simulink library "LSSFunctionLibrary"  (R2019b)
settings: Solver=ode1  StartTime=0.0  StopTime=Inf  FixedStep=0.001  RelTol=1e-3  EnableMultiTasking=on
PostLoadFcn:
  | , if any(exist('dsrtsu_mdlpostloadfcn', 'file') == [2, 3, 6]), try dsrtsu_mdlpostloadfcn('Execute', bdroot); catch fprintf('Error in PostLoadFcn (dsrtsu_mdlpostloadfcn) for model "%s":\n %s\n', bdroot, lasterr); end, end,
undefined symbols (not defined in the file): P_A1_comp_max, P_allow_lane_center_fade, P_assumed_lane_width, P_enable_A1_comp, P_invalid_lane_width_jump_limit, P_Lane_A0_Conf_Limit, P_LCC_STC_AntiWindup_Limit, P_long_dist_camera_to_tire, P_Max_Lane_Width
libraries: $bdroot x1, simulink x1
settings Model: DSRTSU_INTERNAL_RTI_VER=500  DSRTSU_INTERNAL_RTI_TYPE=rti1401  TLRevision=101  RTICANMMDATA=struct('GeneralSetupData',struct('modelroot','C:\WORK\34_GAC\3_A12\A12_H_P\CS322\99999088_GAC_A12P_L2P_Feature_Release\GAC_A12P\DelphiCoreLib\Lateral_Control\ELK','generalsettings',struct('filesettings',struct('destfolder',struct('Name','RTICANMM_FILES','Check',1),'buildfolder',struct('Name','.','Check',1),'AbsDestfolder',struct('Name','C:\WORK\34_GAC\3_A12\A12_H_P\CS322\99999088_GAC_A12P_L2P_Feature_Release\GAC_A12P\DelphiCoreLib\Lateral_Control\ELK\RTICANMM_FILES'),'AbsBuildfolder',struct('Name','C:\WORK\34_GAC\3_A12\A12_H_P\CS322\99999088_GAC_A12P_L2P_Feature_Release\GAC_A12P\DelphiCoreLib\Lateral_Control\ELK'))),'options',struct('addpaths',1,'rmpaths',1,'addtrcexclusion',logical(1),'cannavigator',struct('checkmonitoring',0),'show_usrtrc',0,'use_usrtrc',0),'advanced',struct('options',ones(1,100)),'MPSetup',{{}},'modelname','ELK_fcns_lib','block','ELK_fcns_lib'))  DSRTSU_INTERNAL_RTIFLEXRAYCONFIG=110  DSRTSU_INTERNAL_RTIFPGA=90  Creator=bzxk5y  LastModifiedBy=86156
settings DataIOCC: LimitDataPoints=on  SaveFormat=Array  SignalLoggingSaveFormat=ModelDataLogs  ReturnWorkspaceOutputs=off
settings OptimizationCC: BlockReduction=off  OptimizeBlockIOStorage=off  BufferReuse=off  GlobalBufferReuse=off  ExpressionFolding=off  ExpressionDepthLimit=2147483647  LocalBlockOutputs=off  LifeSpan=inf
settings DebuggingCC: UnderspecifiedInitializationDetection=Classic  MergeDetectMultiDrivingBlocksExec=none  SolverPrmCheckMsg=warning  FcnCallInpInsideContextMsg=warning  AllowSymbolicDim=off  StateNameClashWarn=warning  SFUnexpectedBacktrackingDiag=warning  SFNoUnconditionalDefaultTransitionDiag=warning  SFExecutionAtInitializationDiag=none  ArithmeticOperatorsInVariantConditions=warning
settings HardwareCC: ProdBitPerPointer=32  ProdBitPerSizeT=32  ProdBitPerPtrDiffT=32  ProdLargestAtomicFloat=None  ProdEndianess=BigEndian  ProdWordSize=32  ProdHWDeviceType=Generic->Custom  TargetIntDivRoundTo=Zero  TargetEndianess=BigEndian  TargetHWDeviceType=Generic->Custom
settings ModelReferenceCC: PropagateSignalLabelsOutOfModel=off
settings SFSimCC: SimUseLocalCustomCode=off  CustomCodeUndefinedFunction=UseInterfaceOnly
settings RTWCC: Description=dSPACE DS1401 Hardware Platform  SystemTargetFile=rti1401.tlc  MakeCommand=make_rti  TemplateMakefile=rti1401.tmf  RTWUseLocalCustomCode=off
settings CodeAppCC: StateflowObjectComments=on
settings STFCustomTargetCC: ParMdlRefBuildCompliant=on  MatFileLogging=on  CPPClassGenCompliant=on  SystemTargetFile=rti1401.tlc
settings GRTTargetCC: TargetLangStandard=C89/C90 (ANSI)  CompOptLevelCompliant=off  ConcurrentExecutionCompliant=off  CombineOutputUpdateFcns=off  UseToolchainInfoCompliant=off  ExtModeMexFile=noextcomm
settings ConfigComp: CovMetricSettings=dw  CovSaveCumulativeToWorkspaceVar=on  CovSaveSingleToWorkspaceVar=on  CovExternalEMLEnable=off

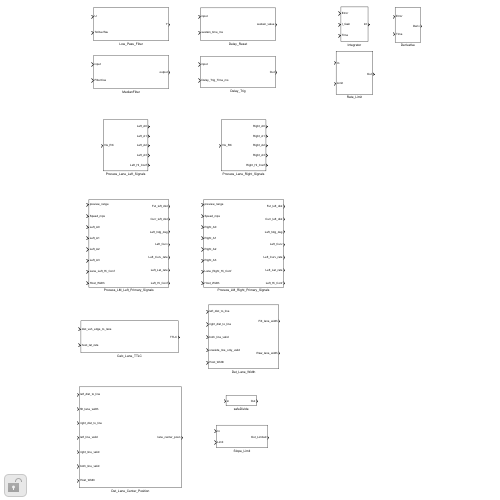
[thumbnail: Simulink's stored preview of the top-level diagram]
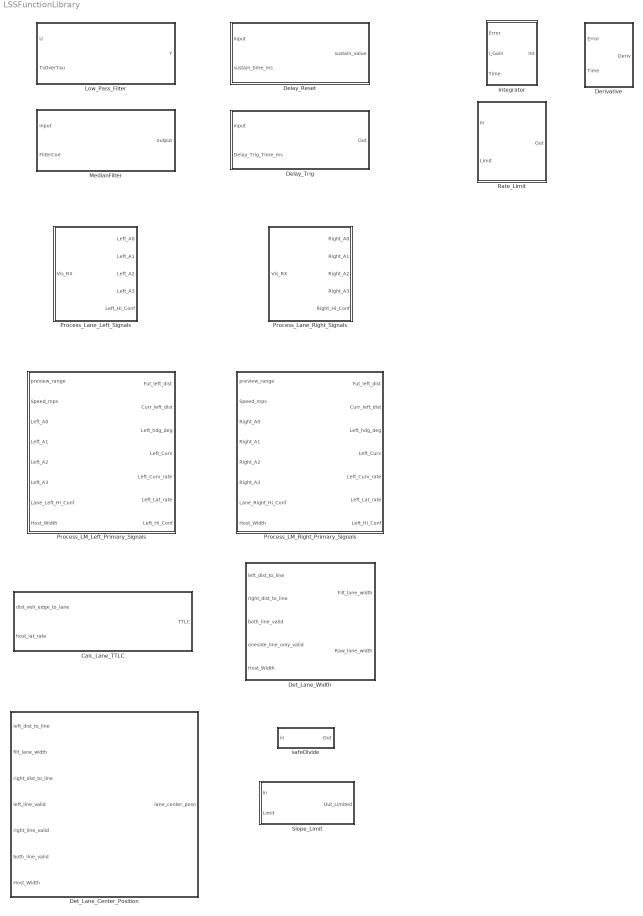
== system LSSFunctionLibrary ==
  Calc_Lane_TTLC : Subsystem
  Delay_Reset : Subsystem
  Delay_Trig : Subsystem
  Derivative : Subsystem
  Det_Lane_Center_Position : Subsystem
  Det_Lane_Width : Subsystem
  Integrator : Subsystem
  Low_Pass_Filter : Subsystem
  MedianFilter : Subsystem
  Process_LM_Left_Primary_Signals : Subsystem
  Process_LM_Right_Primary_Signals : Subsystem
  Process_Lane_Left_Signals : Subsystem
  Process_Lane_Right_Signals : Subsystem
  Rate_Limit : Subsystem
  Slope_Limit : Subsystem
  safeDivide : Subsystem

== system LSSFunctionLibrary/Calc_Lane_TTLC ==
  dist_veh_edge_to_lane : Inport  OutDataTypeStr=single
  host_lat_rate : Inport  Port=2  OutDataTypeStr=single
  Constant : Constant  Value=0.001  OutDataTypeStr=single
  Divide : Product  Inputs=*/  OutDataTypeStr=single
  Max : MinMax  Function=max  Inputs=2  OutDataTypeStr=single
  Saturation : Saturate  UpperLimit=10  LowerLimit=0  OutDataTypeStr=single
  TTLC : Outport  OutDataTypeStr=single
  wires:
  dist_veh_edge_to_lane/1 -> Divide/1
  Max/1 -> Divide/2
  host_lat_rate/1 -> Max/1
  Constant/1 -> Max/2
  Divide/1 -> Saturation/1
  Saturation/1 -> TTLC/1

== system LSSFunctionLibrary/Delay_Reset ==
  input : Inport  Description=_GWMAB30P4.LKAFN.000_316_
  sustain_time_ms : Inport  Description=_GWMAB30P4.LKAFN.000_317_  Port=2
  Sustain_wo_reset : Stateflow chart  Description=_GWMAB30P4.LKAFN.000_319_  TreatAsAtomicUnit=on
  sustain_value : Outport  Description=_GWMAB30P4.LKAFN.000_323_
  wires:
  Sustain_wo_reset/1(sustain_value) -> sustain_value/1
  input/1 -> Sustain_wo_reset/1(input)
  sustain_time_ms/1 -> Sustain_wo_reset/2(sustain_time)

== system LSSFunctionLibrary/Delay_Trig ==
  input : Inport  Description=_GWMAB30P4.LKAFN.000_316_
  Delay_Trig_Time_ms : Inport  Description=_GWMH9P3.LCKFN.000_19_  Port=2
  Delay_Trig : Stateflow chart  TreatAsAtomicUnit=on
  Out : Outport  Description=_GWMH9P3.LCKFN.000_23_
  wires:
  input/1 -> Delay_Trig/1(Input)
  Delay_Trig_Time_ms/1 -> Delay_Trig/2(Delay_Trig_Time)
  Delay_Trig/1(Delay_Trig) -> Out/1

== system LSSFunctionLibrary/Derivative ==
  Error : Inport
  Time : Inport  Port=2
  Delay : Delay  DelayLength=1  InitialCondition=0
  Divide : Product  Inputs=*/
  Sum3 : Sum  Inputs=+-
  Deriv : Outport
  wires:
  Sum3/1 -> Divide/1
  Error/1 -> Delay/1, Sum3/1
  Divide/1 -> Deriv/1  "STC_Error_Derivative"
  Delay/1 -> Sum3/2
  Time/1 -> Divide/2

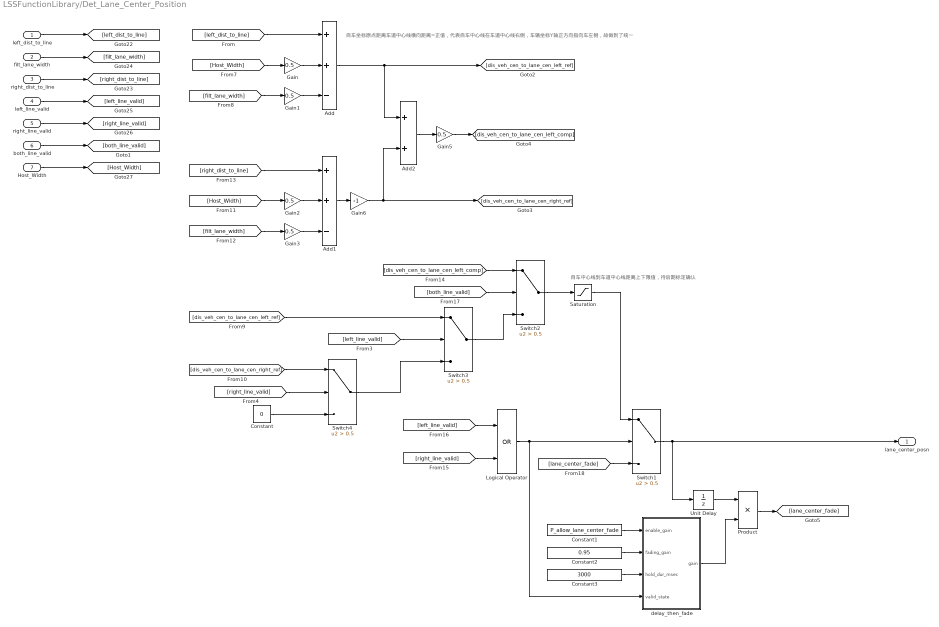
== system LSSFunctionLibrary/Det_Lane_Center_Position ==
  note: 自车中心线到车道中心线距离上下限值，待后期标定确认
  note: 自车坐标原点距离车道中心线横向距离=正值，代表自车中心线在车道中心线右侧，车辆坐标Y轴正方向指向车左侧，故做到了统一
  left_dist_to_line : Inport  OutDataTypeStr=single
  filt_lane_width : Inport  Port=2  OutDataTypeStr=single
  right_dist_to_line : Inport  Port=3  OutDataTypeStr=single
  left_line_valid : Inport  Port=4
  right_line_valid : Inport  Port=5
  both_line_valid : Inport  Port=6
  Host_Width : Inport  Port=7  OutDataTypeStr=single
  Add : Sum  Inputs=++-  OutDataTypeStr=single  AccumDataTypeStr=single
  Add1 : Sum  Inputs=++-  OutDataTypeStr=single  AccumDataTypeStr=single
  Add2 : Sum  OutDataTypeStr=single  AccumDataTypeStr=single
  Constant : Constant  Value=0  OutDataTypeStr=single
  Constant1 : Constant  Value=P_allow_lane_center_fade  OutDataTypeStr=single
  Constant2 : Constant  Value=0.95  OutDataTypeStr=double
  Constant3 : Constant  Value=3000  OutDataTypeStr=single
  Gain{,1..3,5} (5 alike) : Gain  Gain=0.5  OutDataTypeStr=single
  Gain6 : Gain  Gain=-1  OutDataTypeStr=single
  Logical Operator : Logic  Operator=OR  AllPortsSameDT=off  OutDataTypeStr=boolean
  Product : Product  OutDataTypeStr=single
  Saturation : Saturate  UpperLimit=3.5  LowerLimit=-3.5  OutDataTypeStr=single
  Switch{1..4} (4 alike) : Switch  Criteria=u2 > Threshold  Threshold=0.5  OutDataTypeStr=single
  Unit Delay : UnitDelay  SampleTime=-1  HasFrameUpgradeWarning=on
  delay_then_fade : Stateflow chart  TreatAsAtomicUnit=on
  lane_center_posn : Outport  OutDataTypeStr=single
  wires:
  left_dist_to_line/1 -> [left_dist_to_line]
  filt_lane_width/1 -> [filt_lane_width]
  right_dist_to_line/1 -> [right_dist_to_line]
  left_line_valid/1 -> [left_line_valid]
  right_line_valid/1 -> [right_line_valid]
  Host_Width/1 -> [Host_Width]
  [left_dist_to_line] -> Add/1
  both_line_valid/1 -> [both_line_valid]
  [Host_Width] -> Gain/1
  Gain/1 -> Add/2
  Gain1/1 -> Add/3
  [filt_lane_width] -> Gain1/1
  Gain3/1 -> Add1/3
  Gain2/1 -> Add1/2
  [Host_Width] -> Gain2/1
  [right_dist_to_line] -> Add1/1
  [filt_lane_width] -> Gain3/1
  Add/1 -> Add2/1, [dis_veh_cen_to_lane_cen_left_ref]
  Add1/1 -> Gain6/1
  Add2/1 -> Gain5/1
  Gain5/1 -> [dis_veh_cen_to_lane_cen_left_comp]
  [left_line_valid] -> Logical Operator/1
  [right_line_valid] -> Logical Operator/2
  [both_line_valid] -> Switch2/2
  Switch2/1 -> Saturation/1
  [dis_veh_cen_to_lane_cen_left_comp] -> Switch2/1
  Switch3/1 -> Switch2/3
  [left_line_valid] -> Switch3/2
  [dis_veh_cen_to_lane_cen_left_ref] -> Switch3/1
  Switch4/1 -> Switch3/3
  [right_line_valid] -> Switch4/2
  [dis_veh_cen_to_lane_cen_right_ref] -> Switch4/1
  Constant/1 -> Switch4/3
  Switch1/1 -> Unit Delay/1, lane_center_posn/1
  Constant1/1 -> delay_then_fade/1(enable_gain)
  Constant2/1 -> delay_then_fade/2(fading_gain)
  Constant3/1 -> delay_then_fade/3(hold_dur_msec)
  Logical Operator/1 -> delay_then_fade/4(valid_state), Switch1/2
  Unit Delay/1 -> Product/1
  delay_then_fade/1(gain) -> Product/2
  Product/1 -> [lane_center_fade]
  [lane_center_fade] -> Switch1/3
  Saturation/1 -> Switch1/1
  Gain6/1 -> Add2/2, [dis_veh_cen_to_lane_cen_right_ref]

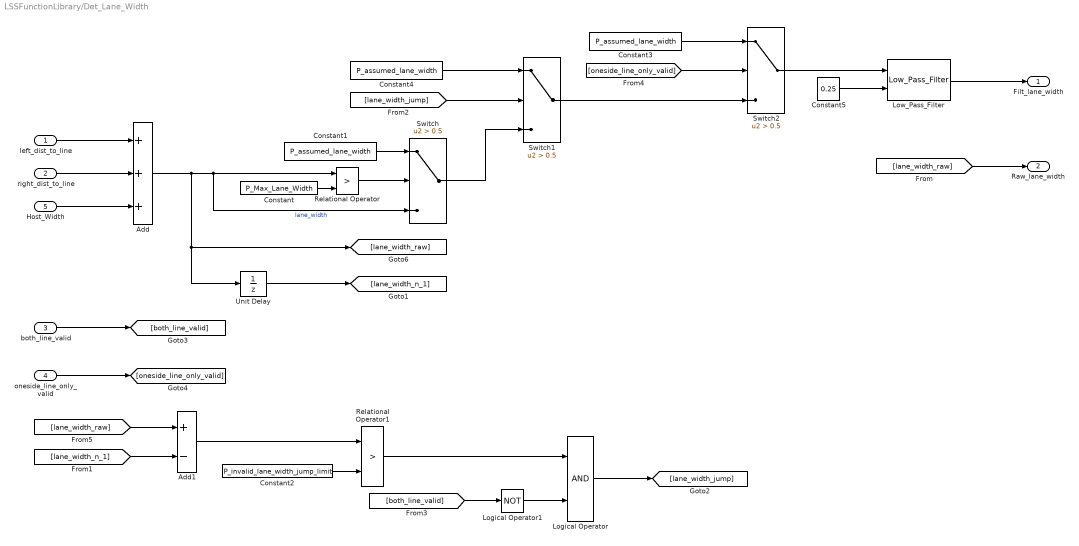
== system LSSFunctionLibrary/Det_Lane_Width ==
  left_dist_to_line : Inport  OutDataTypeStr=single
  right_dist_to_line : Inport  Port=2  OutDataTypeStr=single
  both_line_valid : Inport  Port=3
  oneside_line_only_valid : Inport  Port=4
  Host_Width : Inport  Port=5  OutDataTypeStr=single
  Add : Sum  Inputs=+++  OutDataTypeStr=single  AccumDataTypeStr=single
  Add1 : Sum  Inputs=+-  OutDataTypeStr=single  AccumDataTypeStr=single
  Constant : Constant  Value=P_Max_Lane_Width  OutDataTypeStr=single
  Constant1 : Constant  Value=P_assumed_lane_width  OutDataTypeStr=single
  Constant2 : Constant  Value=P_invalid_lane_width_jump_limit  OutDataTypeStr=single
  Constant3 : Constant  Value=P_assumed_lane_width  OutDataTypeStr=single
  Constant4 : Constant  Value=P_assumed_lane_width  OutDataTypeStr=single
  Constant5 : Constant  Value=0.25  OutDataTypeStr=single
  Logical Operator : Logic  AllPortsSameDT=off  OutDataTypeStr=boolean
  Logical Operator1 : Logic  Operator=NOT  AllPortsSameDT=off  OutDataTypeStr=boolean
  Low_Pass_Filter : $bdroot/Low_Pass_Filter  SystemSampleTime=-1  Latency=0  AutoFrameSizeCalculation=off
  Relational Operator : RelationalOperator  Operator=>  OutDataTypeStr=boolean  RndMeth=Simplest
  Relational Operator1 : RelationalOperator  Operator=>  OutDataTypeStr=boolean  RndMeth=Simplest
  Switch : Switch  Criteria=u2 > Threshold  Threshold=0.5  OutDataTypeStr=single
  Switch1 : Switch  Criteria=u2 > Threshold  Threshold=0.5  OutDataTypeStr=single
  Switch2 : Switch  Criteria=u2 > Threshold  Threshold=0.5  OutDataTypeStr=single
  Unit Delay : UnitDelay  SampleTime=-1  HasFrameUpgradeWarning=on
  Filt_lane_width : Outport  OutDataTypeStr=single
  Raw_lane_width : Outport  Port=2  OutDataTypeStr=single
  wires:
  right_dist_to_line/1 -> Add/2
  left_dist_to_line/1 -> Add/1
  Host_Width/1 -> Add/3
  Add/1 -> Unit Delay/1, [lane_width_raw], Switch/3, Relational Operator/1  "lane_width"
  Constant/1 -> Relational Operator/2
  Relational Operator/1 -> Switch/2
  Constant1/1 -> Switch/1
  Unit Delay/1 -> [lane_width_n_1]
  [lane_width_raw] -> Add1/1
  [lane_width_n_1] -> Add1/2
  Add1/1 -> Relational Operator1/1
  Constant2/1 -> Relational Operator1/2
  Relational Operator1/1 -> Logical Operator/1
  Logical Operator1/1 -> Logical Operator/2
  Logical Operator/1 -> [lane_width_jump]
  [lane_width_jump] -> Switch1/2
  Switch/1 -> Switch1/3
  both_line_valid/1 -> [both_line_valid]
  oneside_line_only_valid/1 -> [oneside_line_only_valid]
  [both_line_valid] -> Logical Operator1/1
  [oneside_line_only_valid] -> Switch2/2
  Switch1/1 -> Switch2/3
  Constant3/1 -> Switch2/1
  Constant4/1 -> Switch1/1
  Switch2/1 -> Low_Pass_Filter/1
  Constant5/1 -> Low_Pass_Filter/2
  Low_Pass_Filter/1 -> Filt_lane_width/1
  [lane_width_raw] -> Raw_lane_width/1

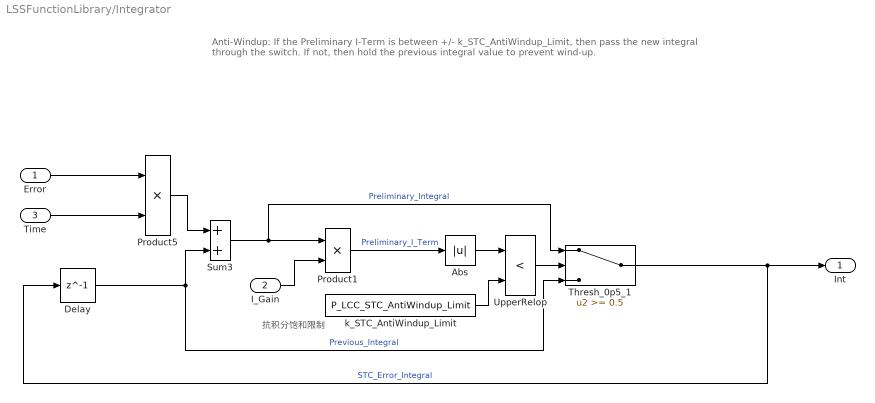
== system LSSFunctionLibrary/Integrator ==
  note: 抗积分饱和限制
  note: Anti-Windup:
      | 	If the Preliminary I-Term is between +/- k_STC_AntiWindup_Limit, then pass the new integral through the switch.
      | 	If not, then hold the previous integral value to prevent wind-up.
  Error : Inport
  I_Gain : Inport  Port=2
  Time : Inport  Port=3
  Abs : Abs
  Delay : Delay  DelayLength=1  InitialCondition=0
  Product1 : Product
  Product5 : Product
  Sum3 : Sum
  Thresh_0p5_1 : Switch  Threshold=0.5
  UpperRelop : RelationalOperator  DisableCoverage=on  Operator=<  OutDataTypeStr=boolean  RndMeth=Nearest
  k_STC_AntiWindup_Limit : Constant  Value=P_LCC_STC_AntiWindup_Limit  OutDataTypeStr=single
  Int : Outport
  wires:
  Time/1 -> Product5/2
  Product5/1 -> Sum3/1
  Delay/1 -> Sum3/2, Thresh_0p5_1/3  "Previous_Integral"
  Error/1 -> Product5/1
  Thresh_0p5_1/1 -> Int/1, Delay/1  "STC_Error_Integral"
  Sum3/1 -> Product1/1, Thresh_0p5_1/1  "Preliminary_Integral"
  I_Gain/1 -> Product1/2
  Product1/1 -> Abs/1  "Preliminary_I_Term"
  Abs/1 -> UpperRelop/1
  k_STC_AntiWindup_Limit/1 -> UpperRelop/2
  UpperRelop/1 -> Thresh_0p5_1/2

== system LSSFunctionLibrary/Low_Pass_Filter ==
  note: y_n-1
  note: y_(n) = w*T*(u_n - y_(n-1)) - y_(n-1)
  U : Inport
      settings: AttributesFormatString=DT=%<OutDataTypeStr>
  TsOverTau : Inport  Port=2
      settings: AttributesFormatString=DT=%<OutDataTypeStr>
  S16_Lag_Filter : Subsystem
  UD_1 : UnitDelay  Description=_3p1p0.CLib.000_109_  SampleTime=-1  HasFrameUpgradeWarning=on
  Y : Outport
      settings: AttributesFormatString=DT=%<OutDataTypeStr>
  wires:
  U/1 -> S16_Lag_Filter/1(unfiltered_input)  "U"
  TsOverTau/1 -> S16_Lag_Filter/3(filter_gain)  "TsOverTau"
  UD_1/1 -> S16_Lag_Filter/2(filtered_value_n_1)  "LastY"
  S16_Lag_Filter/1(filtered_output) -> Y/1, UD_1/1  "Y"

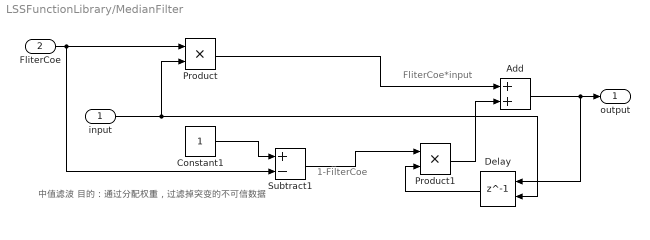
== system LSSFunctionLibrary/MedianFilter ==
  note: FliterCoe*input
  note: 1-FilterCoe
  note: 中值滤波
      | 目的：通过分配权重，过滤掉突变的不可信数据
  input : Inport
  FliterCoe : Inport  Port=2
  Add : Sum
  Constant1 : Constant  OutDataTypeStr=single
  Delay : Delay  DelayLength=1  InitialConditionSource=Input port
      settings: InputPortMap=u0,p4
  Product : Product
  Product1 : Product
  Subtract1 : Sum  Inputs=+-
  output : Outport
  wires:
  Product1/1 -> Add/2
  input/1 -> Product/2, Delay/2
  Constant1/1 -> Subtract1/1
  Delay/1 -> Product1/2
  FliterCoe/1 -> Product/1, Subtract1/2
  Product/1 -> Add/1
  Add/1 -> Delay/1, output/1
  Subtract1/1 -> Product1/1

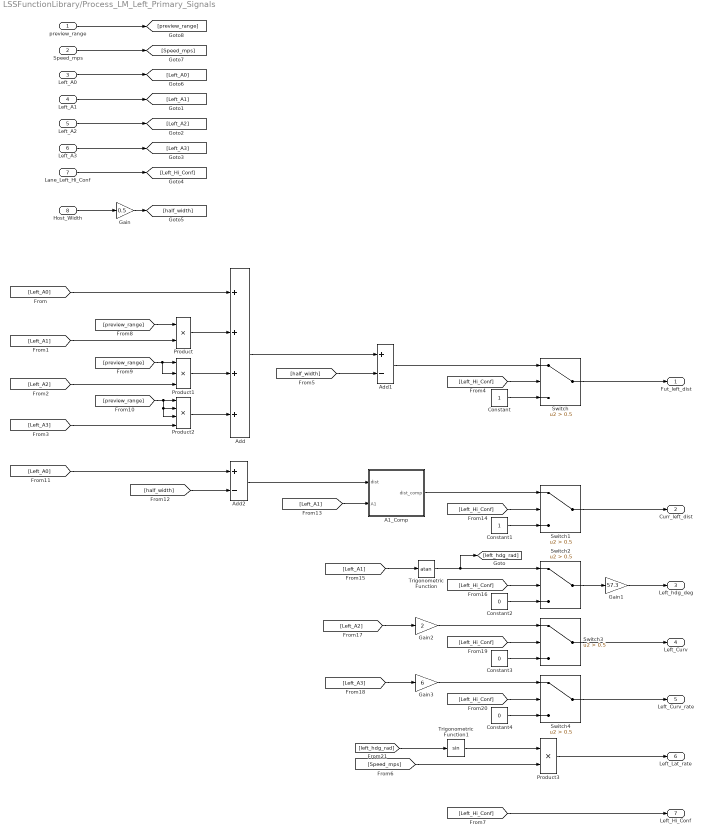
== system LSSFunctionLibrary/Process_LM_Left_Primary_Signals ==
  preview_range : Inport  OutDataTypeStr=single
  Speed_mps : Inport  Port=2  OutDataTypeStr=single
  Left_A0 : Inport  Port=3  OutDataTypeStr=single
  Left_A1 : Inport  Port=4  OutDataTypeStr=single
  Left_A2 : Inport  Port=5  OutDataTypeStr=single
  Left_A3 : Inport  Port=6  OutDataTypeStr=single
  Lane_Left_Hi_Conf : Inport  Port=7  OutDataTypeStr=boolean
  Host_Width : Inport  Port=8  OutDataTypeStr=single
  A1_Comp : Subsystem
  Add : Sum  Inputs=++++  OutDataTypeStr=single  AccumDataTypeStr=single
  Add1 : Sum  Inputs=+-  OutDataTypeStr=single  AccumDataTypeStr=single
  Add2 : Sum  Inputs=+-  OutDataTypeStr=single  AccumDataTypeStr=single
  Constant : Constant
  Constant1 : Constant
  Constant2 : Constant  Value=0
  Constant3 : Constant  Value=0
  Constant4 : Constant  Value=0
  Gain : Gain  Gain=0.5  OutDataTypeStr=single
  Gain1 : Gain  Gain=57.3  OutDataTypeStr=single
  Gain2 : Gain  Gain=2  OutDataTypeStr=single
  Gain3 : Gain  Gain=6  OutDataTypeStr=single
  Product : Product  OutDataTypeStr=single
  Product1 : Product  Inputs=3  OutDataTypeStr=single
  Product2 : Product  Inputs=4  OutDataTypeStr=single
  Product3 : Product  OutDataTypeStr=single
  Switch{,1..4} (5 alike) : Switch  Criteria=u2 > Threshold  Threshold=0.5  OutDataTypeStr=single
  Trigonometric Function : Trigonometry  Operator=atan
  Trigonometric Function1 : Trigonometry
  Fut_left_dist : Outport  OutDataTypeStr=single
  Curr_left_dist : Outport  Port=2  OutDataTypeStr=single
  Left_hdg_deg : Outport  Port=3  OutDataTypeStr=single
  Left_Curv : Outport  Port=4  OutDataTypeStr=single
  Left_Curv_rate : Outport  Port=5  OutDataTypeStr=single
  Left_Lat_rate : Outport  Port=6  OutDataTypeStr=single
  Left_Hi_Conf : Outport  Port=7
  wires:
  Left_A3/1 -> [Left_A3]
  Lane_Left_Hi_Conf/1 -> [Left_Hi_Conf]
  Left_A2/1 -> [Left_A2]
  Left_A1/1 -> [Left_A1]
  Left_A0/1 -> [Left_A0]
  Host_Width/1 -> Gain/1
  Gain/1 -> [half_width]
  Speed_mps/1 -> [Speed_mps]
  preview_range/1 -> [preview_range]
  [Left_A0] -> Add/1
  [preview_range] -> Product/1
  [Left_A1] -> Product/2
  Product/1 -> Add/2
  [preview_range] -> Product1/2, Product1/1
  [Left_A2] -> Product1/3
  Product1/1 -> Add/3
  [Left_A3] -> Product2/4
  [preview_range] -> Product2/3, Product2/2, Product2/1
  Product2/1 -> Add/4
  [Left_Hi_Conf] -> Switch/2
  Constant/1 -> Switch/3
  [half_width] -> Add1/2
  Add/1 -> Add1/1
  Add1/1 -> Switch/1
  Switch/1 -> Fut_left_dist/1
  Add2/1 -> A1_Comp/1(dist)
  [half_width] -> Add2/2
  [Left_A0] -> Add2/1
  [Left_A1] -> A1_Comp/2(A1)
  Switch1/1 -> Curr_left_dist/1
  A1_Comp/1(dist_comp) -> Switch1/1
  Constant1/1 -> Switch1/3
  [Left_Hi_Conf] -> Switch1/2
  [Left_A1] -> Trigonometric Function/1
  Switch2/1 -> Gain1/1
  Trigonometric Function/1 -> [left_hdg_rad], Switch2/1
  Constant2/1 -> Switch2/3
  [Left_Hi_Conf] -> Switch2/2
  Gain1/1 -> Left_hdg_deg/1
  [Left_A2] -> Gain2/1
  [Left_A3] -> Gain3/1
  [Left_Hi_Conf] -> Switch3/2
  Constant3/1 -> Switch3/3
  Gain2/1 -> Switch3/1
  Switch3/1 -> Left_Curv/1
  Switch4/1 -> Left_Curv_rate/1
  Gain3/1 -> Switch4/1
  Constant4/1 -> Switch4/3
  [Left_Hi_Conf] -> Switch4/2
  [left_hdg_rad] -> Trigonometric Function1/1
  Trigonometric Function1/1 -> Product3/1
  [Speed_mps] -> Product3/2
  Product3/1 -> Left_Lat_rate/1
  [Left_Hi_Conf] -> Left_Hi_Conf/1

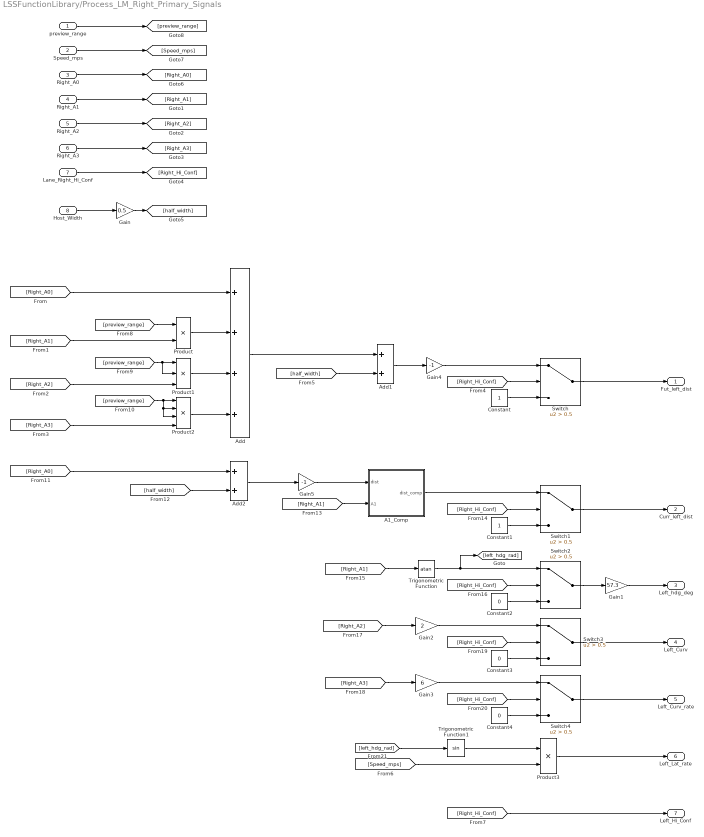
== system LSSFunctionLibrary/Process_LM_Right_Primary_Signals ==
  preview_range : Inport  OutDataTypeStr=single
  Speed_mps : Inport  Port=2  OutDataTypeStr=single
  Right_A0 : Inport  Port=3  OutDataTypeStr=single
  Right_A1 : Inport  Port=4  OutDataTypeStr=single
  Right_A2 : Inport  Port=5  OutDataTypeStr=single
  Right_A3 : Inport  Port=6  OutDataTypeStr=single
  Lane_Right_Hi_Conf : Inport  Port=7  OutDataTypeStr=boolean
  Host_Width : Inport  Port=8  OutDataTypeStr=single
  A1_Comp : Subsystem
  Add : Sum  Inputs=++++  OutDataTypeStr=single  AccumDataTypeStr=single
  Add1 : Sum  AccumDataTypeStr=single
  Add2 : Sum  OutDataTypeStr=single  AccumDataTypeStr=single
  Constant : Constant
  Constant1 : Constant
  Constant2 : Constant  Value=0
  Constant3 : Constant  Value=0
  Constant4 : Constant  Value=0
  Gain : Gain  Gain=0.5  OutDataTypeStr=single
  Gain1 : Gain  Gain=57.3  OutDataTypeStr=single
  Gain2 : Gain  Gain=2  OutDataTypeStr=single
  Gain3 : Gain  Gain=6  OutDataTypeStr=single
  Gain4 : Gain  Gain=-1  OutDataTypeStr=single
  Gain5 : Gain  Gain=-1  OutDataTypeStr=single
  Product : Product  OutDataTypeStr=single
  Product1 : Product  Inputs=3  OutDataTypeStr=single
  Product2 : Product  Inputs=4  OutDataTypeStr=single
  Product3 : Product  OutDataTypeStr=single
  Switch{,1..4} (5 alike) : Switch  Criteria=u2 > Threshold  Threshold=0.5  OutDataTypeStr=single
  Trigonometric Function : Trigonometry  Operator=atan
  Trigonometric Function1 : Trigonometry
  Fut_left_dist : Outport  OutDataTypeStr=single
  Curr_left_dist : Outport  Port=2  OutDataTypeStr=single
  Left_hdg_deg : Outport  Port=3  OutDataTypeStr=single
  Left_Curv : Outport  Port=4  OutDataTypeStr=single
  Left_Curv_rate : Outport  Port=5  OutDataTypeStr=single
  Left_Lat_rate : Outport  Port=6  OutDataTypeStr=single
  Left_Hi_Conf : Outport  Port=7  OutDataTypeStr=boolean
  wires:
  [Right_Hi_Conf] -> Left_Hi_Conf/1
  Product3/1 -> Left_Lat_rate/1
  [Speed_mps] -> Product3/2
  Trigonometric Function1/1 -> Product3/1
  [left_hdg_rad] -> Trigonometric Function1/1
  [Right_Hi_Conf] -> Switch4/2
  Constant4/1 -> Switch4/3
  Gain3/1 -> Switch4/1
  Switch4/1 -> Left_Curv_rate/1
  Switch3/1 -> Left_Curv/1
  Gain2/1 -> Switch3/1
  Constant3/1 -> Switch3/3
  [Right_Hi_Conf] -> Switch3/2
  [Right_A3] -> Gain3/1
  [Right_A2] -> Gain2/1
  Gain1/1 -> Left_hdg_deg/1
  [Right_Hi_Conf] -> Switch2/2
  Constant2/1 -> Switch2/3
  Trigonometric Function/1 -> Switch2/1, [left_hdg_rad]
  Switch2/1 -> Gain1/1
  [Right_A1] -> Trigonometric Function/1
  [Right_Hi_Conf] -> Switch1/2
  Constant1/1 -> Switch1/3
  A1_Comp/1(dist_comp) -> Switch1/1
  Switch1/1 -> Curr_left_dist/1
  [Right_A1] -> A1_Comp/2(A1)
  [Right_A0] -> Add2/1
  [half_width] -> Add2/2
  Add2/1 -> Gain5/1
  Switch/1 -> Fut_left_dist/1
  Add1/1 -> Gain4/1
  Add/1 -> Add1/1
  [half_width] -> Add1/2
  Constant/1 -> Switch/3
  [Right_Hi_Conf] -> Switch/2
  Product2/1 -> Add/4
  [preview_range] -> Product2/1, Product2/2, Product2/3
  [Right_A3] -> Product2/4
  Product1/1 -> Add/3
  [Right_A2] -> Product1/3
  [preview_range] -> Product1/1, Product1/2
  Product/1 -> Add/2
  [Right_A1] -> Product/2
  [preview_range] -> Product/1
  [Right_A0] -> Add/1
  preview_range/1 -> [preview_range]
  Speed_mps/1 -> [Speed_mps]
  Gain/1 -> [half_width]
  Host_Width/1 -> Gain/1
  Right_A0/1 -> [Right_A0]
  Right_A1/1 -> [Right_A1]
  Right_A2/1 -> [Right_A2]
  Lane_Right_Hi_Conf/1 -> [Right_Hi_Conf]
  Right_A3/1 -> [Right_A3]
  Gain4/1 -> Switch/1
  Gain5/1 -> A1_Comp/1(dist)

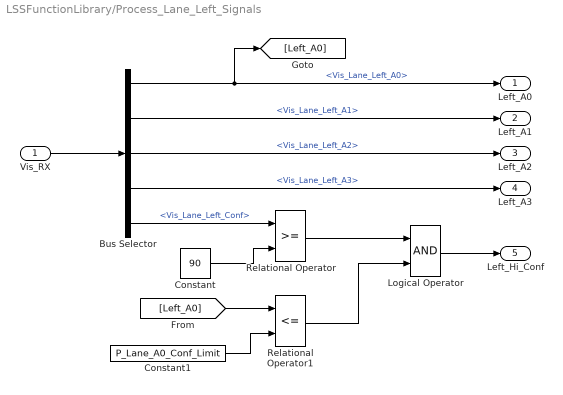
== system LSSFunctionLibrary/Process_Lane_Left_Signals ==
  Vis_RX : Inport  OutDataTypeStr=single
  Bus Selector : BusSelector  OutputSignals=Vis_Lane_Left_A0,Vis_Lane_Left_A1,Vis_Lane_Left_A2,Vis_Lane_Left_A3,Vis_Lane_Left_Conf
  Constant : Constant  Value=90  OutDataTypeStr=single
  Constant1 : Constant  Value=P_Lane_A0_Conf_Limit  OutDataTypeStr=single
  Logical Operator : Logic  AllPortsSameDT=off  OutDataTypeStr=boolean
  Relational Operator : RelationalOperator  OutDataTypeStr=boolean  RndMeth=Simplest
  Relational Operator1 : RelationalOperator  Operator=<=  OutDataTypeStr=boolean  RndMeth=Simplest
  Left_A0 : Outport  OutDataTypeStr=single
  Left_A1 : Outport  Port=2  OutDataTypeStr=single
  Left_A2 : Outport  Port=3  OutDataTypeStr=single
  Left_A3 : Outport  Port=4  OutDataTypeStr=single
  Left_Hi_Conf : Outport  Port=5  OutDataTypeStr=boolean
  wires:
  Vis_RX/1 -> Bus Selector/1
  Bus Selector/1 -> [Left_A0], Left_A0/1  "<Vis_Lane_Left_A0>"
  Bus Selector/2 -> Left_A1/1  "<Vis_Lane_Left_A1>"
  Bus Selector/3 -> Left_A2/1  "<Vis_Lane_Left_A2>"
  Bus Selector/4 -> Left_A3/1  "<Vis_Lane_Left_A3>"
  Bus Selector/5 -> Relational Operator/1  "<Vis_Lane_Left_Conf>"
  Constant/1 -> Relational Operator/2
  [Left_A0] -> Relational Operator1/1
  Constant1/1 -> Relational Operator1/2
  Relational Operator/1 -> Logical Operator/1
  Relational Operator1/1 -> Logical Operator/2
  Logical Operator/1 -> Left_Hi_Conf/1

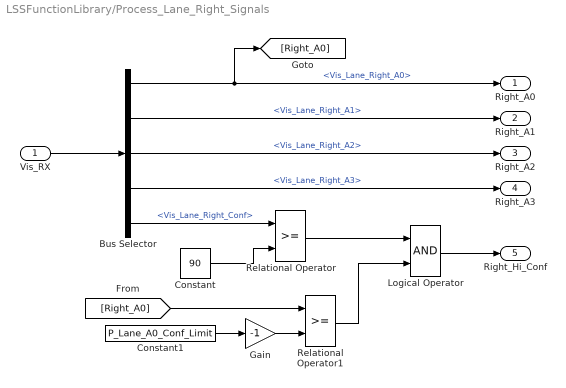
== system LSSFunctionLibrary/Process_Lane_Right_Signals ==
  Vis_RX : Inport  OutDataTypeStr=single
  Bus Selector : BusSelector  OutputSignals=Vis_Lane_Right_A0,Vis_Lane_Right_A1,Vis_Lane_Right_A2,Vis_Lane_Right_A3,Vis_Lane_Right_Conf
  Constant : Constant  Value=90  OutDataTypeStr=single
  Constant1 : Constant  Value=P_Lane_A0_Conf_Limit  OutDataTypeStr=single
  Gain : Gain  Gain=-1  OutDataTypeStr=single
  Logical Operator : Logic  AllPortsSameDT=off  OutDataTypeStr=boolean
  Relational Operator : RelationalOperator  OutDataTypeStr=boolean  RndMeth=Simplest
  Relational Operator1 : RelationalOperator  OutDataTypeStr=boolean  RndMeth=Simplest
  Right_A0 : Outport  OutDataTypeStr=single
  Right_A1 : Outport  Port=2  OutDataTypeStr=single
  Right_A2 : Outport  Port=3  OutDataTypeStr=single
  Right_A3 : Outport  Port=4  OutDataTypeStr=single
  Right_Hi_Conf : Outport  Port=5  OutDataTypeStr=boolean
  wires:
  Logical Operator/1 -> Right_Hi_Conf/1
  Relational Operator1/1 -> Logical Operator/2
  Relational Operator/1 -> Logical Operator/1
  [Right_A0] -> Relational Operator1/1
  Constant/1 -> Relational Operator/2
  Bus Selector/5 -> Relational Operator/1  "<Vis_Lane_Right_Conf>"
  Bus Selector/4 -> Right_A3/1  "<Vis_Lane_Right_A3>"
  Bus Selector/3 -> Right_A2/1  "<Vis_Lane_Right_A2>"
  Bus Selector/2 -> Right_A1/1  "<Vis_Lane_Right_A1>"
  Bus Selector/1 -> Right_A0/1, [Right_A0]  "<Vis_Lane_Right_A0>"
  Vis_RX/1 -> Bus Selector/1
  Constant1/1 -> Gain/1
  Gain/1 -> Relational Operator1/2

== system LSSFunctionLibrary/Rate_Limit ==
  note: U(k)
  note: Y(k-1)
  note: ( U(k) - Y(k-1) )
  note: Y(k-1)
  note: Y(k)
  In : Inport
  Limit : Inport  Port=2
  Delay Input2 : UnitDelay  Description=Store in Global RAM  DisableCoverage=on  SampleTime=-1  HasFrameUpgradeWarning=on
  Difference Inputs1 : Sum  Description=Add in CPU  DisableCoverage=on  Inputs=+-  OutDataTypeStr=Inherit: Inherit via back propagation
  Difference Inputs2 : Sum  Description=Add in CPU  OutDataTypeStr=Inherit: Same as first input
  Gain7 : Gain  Gain=-1  OutDataTypeStr=single
  SaturationDynamic : simulink/Discontinuities/Saturation Dynamic  OutMin=[]  OutMax=[]  OutDataTypeStr=single  OutputDataTypeScalingMode=single  OutDataType=single  OutScaling=2^-10  DoSatur=off
  Out : Outport
  wires:
  Difference Inputs2/1 -> Delay Input2/1, Out/1
  In/1 -> Difference Inputs1/1
  SaturationDynamic/1 -> Difference Inputs2/1
  Gain7/1 -> SaturationDynamic/3
  Limit/1 -> SaturationDynamic/1, Gain7/1
  Difference Inputs1/1 -> SaturationDynamic/2
  Delay Input2/1 -> Difference Inputs1/2, Difference Inputs2/2

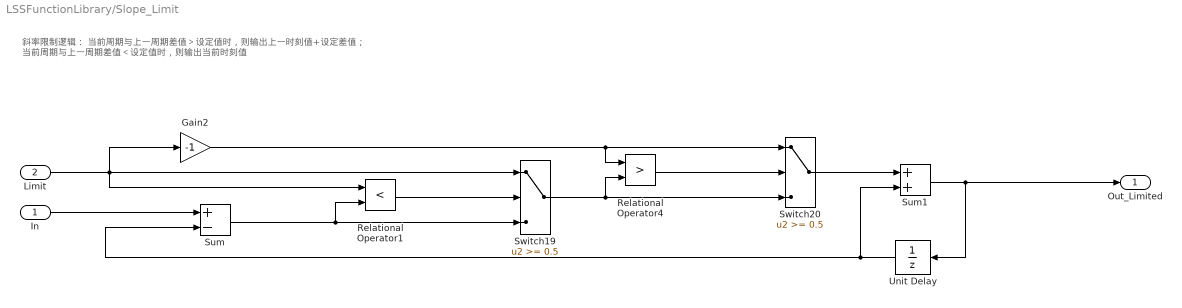
== system LSSFunctionLibrary/Slope_Limit ==
  note: 斜率限制逻辑：
      | 当前周期与上一周期差值＞设定值时，则输出上一时刻值+设定差值；
      | 当前周期与上一周期差值＜设定值时，则输出当前时刻值
  In : Inport
  Limit : Inport  Port=2
  Gain2 : Gain  Description=_GWMH9P2.LKAFN.000_7_  Gain=-1
  Relational Operator1 : RelationalOperator  Description=_GWMH9P2.LKAFN.000_11_  Operator=<  RndMeth=Nearest
  Relational Operator4 : RelationalOperator  Description=_GWMH9P2.LKAFN.000_12_  Operator=>  RndMeth=Nearest
  Sum : Sum  Description=_GWMH9P2.LKAFN.000_13_  Inputs=+-  InputSameDT=on  OutDataTypeStr=Inherit: Same as first input
  Sum1 : Sum  Description=_GWMH9P2.LKAFN.000_14_  InputSameDT=on  OutDataTypeStr=Inherit: Same as first input
  Switch19 : Switch  Description=_GWMH9P2.LKAFN.000_15_  Threshold=0.5  OutDataTypeStr=Inherit: Inherit via back propagation
  Switch20 : Switch  Description=_GWMH9P2.LKAFN.000_16_  Threshold=0.5  OutDataTypeStr=Inherit: Inherit via back propagation
  Unit Delay : UnitDelay  Description=_GWMH9P2.LKAFN.000_17_  SampleTime=-1  HasFrameUpgradeWarning=on
  Out_Limited : Outport
  wires:
  Switch19/1 -> Relational Operator4/2, Switch20/3
  Gain2/1 -> Switch20/1, Relational Operator4/1
  Relational Operator1/1 -> Switch19/2
  In/1 -> Sum/1
  Unit Delay/1 -> Sum/2, Sum1/2
  Switch20/1 -> Sum1/1
  Sum1/1 -> Unit Delay/1, Out_Limited/1
  Relational Operator4/1 -> Switch20/2
  Sum/1 -> Relational Operator1/2, Switch19/3
  Limit/1 -> Gain2/1, Switch19/1, Relational Operator1/1

== system LSSFunctionLibrary/safeDivide ==
  in : Inport  OutDataTypeStr=single
  Abs : Abs  OutDataTypeStr=single
  Constant : Constant  Value=0.000001  OutDataTypeStr=single
  Constant1 : Constant  Value=0.00001  OutDataTypeStr=single
  Relational Operator : RelationalOperator  Operator=>  OutDataTypeStr=boolean  RndMeth=Simplest
  Switch : Switch  Criteria=u2 > Threshold  Threshold=0.5  OutDataTypeStr=single
  Out : Outport  OutDataTypeStr=single
  wires:
  Switch/1 -> Out/1
  Constant/1 -> Relational Operator/2
  Constant1/1 -> Switch/3
  in/1 -> Switch/1, Abs/1
  Relational Operator/1 -> Switch/2
  Abs/1 -> Relational Operator/1

== system LSSFunctionLibrary/Low_Pass_Filter/S16_Lag_Filter ==
  unfiltered_input : Inport
  filtered_value_n_1 : Inport  Port=2
  filter_gain : Inport  Port=3
  Product : Product  Inputs=**  InputSameDT=on  OutDataTypeStr=Inherit: Same as first input
      settings: AttributesFormatString=InputSameDT=%<InputSameDT>
  Product1 : Product  Inputs=**  InputSameDT=on  OutDataTypeStr=Inherit: Same as first input
      settings: AttributesFormatString=InputSameDT=%<InputSameDT>
  Sum1 : Sum  Inputs=-+  InputSameDT=on  OutDataTypeStr=Inherit: Same as first input
      settings: AttributesFormatString=InputSameDT=%<InputSameDT>
  Sum2 : Sum  InputSameDT=on  OutDataTypeStr=Inherit: Same as first input
      settings: AttributesFormatString=InputSameDT=%<InputSameDT>
  filtered_output : Outport
  wires:
  Sum2/1 -> filtered_output/1  "filtered_output"
  Product1/1 -> Sum2/1
  Sum1/1 -> Sum2/2
  Product/1 -> Sum1/1
  filtered_value_n_1/1 -> Product/2, Sum1/2
  filter_gain/1 -> Product1/2, Product/1
  unfiltered_input/1 -> Product1/1

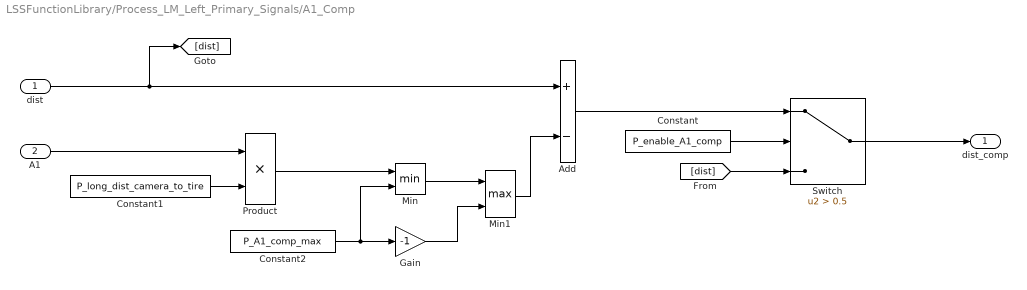
== system LSSFunctionLibrary/Process_LM_Left_Primary_Signals/A1_Comp ==
  dist : Inport  OutDataTypeStr=single
  A1 : Inport  Port=2  OutDataTypeStr=single
  Add : Sum  Inputs=+-  OutDataTypeStr=single  AccumDataTypeStr=single
  Constant : Constant  Value=P_enable_A1_comp  OutDataTypeStr=single
  Constant1 : Constant  Value=P_long_dist_camera_to_tire  OutDataTypeStr=single
  Constant2 : Constant  Value=P_A1_comp_max  OutDataTypeStr=single
  Gain : Gain  Gain=-1  OutDataTypeStr=single
  Min : MinMax  Inputs=2  OutDataTypeStr=single
  Min1 : MinMax  Function=max  Inputs=2  OutDataTypeStr=single
  Product : Product  OutDataTypeStr=single
  Switch : Switch  Criteria=u2 > Threshold  Threshold=0.5  OutDataTypeStr=single
  dist_comp : Outport  OutDataTypeStr=single
  wires:
  dist/1 -> [dist], Add/1
  [dist] -> Switch/3
  Constant/1 -> Switch/2
  Add/1 -> Switch/1
  Switch/1 -> dist_comp/1
  A1/1 -> Product/1
  Constant1/1 -> Product/2
  Product/1 -> Min/1
  Min/1 -> Min1/1
  Min1/1 -> Add/2
  Constant2/1 -> Min/2, Gain/1
  Gain/1 -> Min1/2

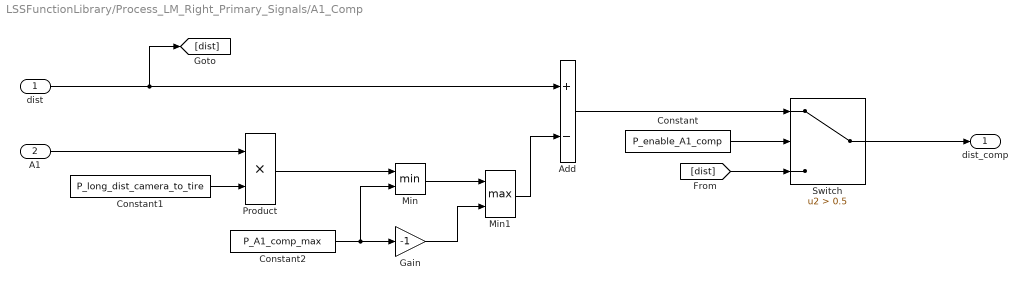
== system LSSFunctionLibrary/Process_LM_Right_Primary_Signals/A1_Comp ==
  dist : Inport  OutDataTypeStr=single
  A1 : Inport  Port=2  OutDataTypeStr=single
  Add : Sum  Inputs=+-  OutDataTypeStr=single  AccumDataTypeStr=single
  Constant : Constant  Value=P_enable_A1_comp  OutDataTypeStr=single
  Constant1 : Constant  Value=P_long_dist_camera_to_tire  OutDataTypeStr=single
  Constant2 : Constant  Value=P_A1_comp_max  OutDataTypeStr=single
  Gain : Gain  Gain=-1  OutDataTypeStr=single
  Min : MinMax  Inputs=2  OutDataTypeStr=single
  Min1 : MinMax  Function=max  Inputs=2  OutDataTypeStr=single
  Product : Product  OutDataTypeStr=single
  Switch : Switch  Criteria=u2 > Threshold  Threshold=0.5  OutDataTypeStr=single
  dist_comp : Outport  OutDataTypeStr=single
  wires:
  Gain/1 -> Min1/2
  Constant2/1 -> Gain/1, Min/2
  Min1/1 -> Add/2
  Min/1 -> Min1/1
  Product/1 -> Min/1
  Constant1/1 -> Product/2
  A1/1 -> Product/1
  Switch/1 -> dist_comp/1
  Add/1 -> Switch/1
  Constant/1 -> Switch/2
  [dist] -> Switch/3
  dist/1 -> Add/1, [dist]

== stateflow chart LSSFunctionLibrary/Delay_Trig/Delay_Trig ==
  settings: description=|
      | _GACA26P4.LCKFN.111_5_
      | $TL$ name=$C_$O; type=Bool; class=default; $TL$
  state OFF
    en: Delay_Trig =0;
    duration= 0;
    settings: description=_GWMH9P5.LCKFN.111_2_
  state ON
    en: Delay_Trig = 0;
    duration=duration+P_LCC_Ts;
    du:duration=duration+P_LCC_Ts;
    settings: description=_GWMH9P5.LCKFN.111_3_
  state Trig
    en: Delay_Trig = 1;
    settings: description=_GWMH9P5.LCKFN.111_4_
  (default) -> OFF
  OFF -> ON : [(Input)]
  ON -> OFF [order 2] : [!Input]
  Trig -> OFF : [!Input]
  ON -> Trig [order 1] : [(Input) && (duration>= Delay_Trig_Time)]
  data: Input input; Delay_Trig_Time input single; Delay_Trig output boolean; duration local single; P_LCC_Ts parameter
  data Input settings: description=_GWMH9P5.LCKFN.111_7_
  data Delay_Trig_Time settings: description=_GWMH9P5.LCKFN.111_8_
  data Delay_Trig settings: description=_GWMH9P5.LCKFN.111_9_
  data duration settings: description=_GWMAB30P3.LCKFN.111_3_$TL$ name=$C_$O; type=Float32; class=default; $TL$

== stateflow chart LSSFunctionLibrary/Det_Lane_Center_Position/delay_then_fade ==
  state standby
    du:
    hold_timer = 0;
    gain = 1;
    settings: description=_GWMH9P4.LKAFN.111_22_
  note: invalid condition
      | starts hold timer
      | where output gain
      | is held at 1
  state hold_gain_for_duration
    en:
    hold_timer = 0;
    du:
    gain = 1;
    hold_timer = hold_timer + Ts;
  note: when hold duration
      | expires, set gain to
      | lower value < 1 (fading_gain)
      | which will recursively
      | bring the abs lane
      | position to zero
      | (abs posn = abs_posn_n_1 * fading_gain)
  state fade_gain
    du:
    gain = fading_gain;
    settings: description=_GWMH9P4.LKAFN.111_20_
  (default) -> standby
  (junction 27) -> standby
  (junction 25) -> (junction 27) : [valid_state > 0.5]
  standby -> hold_gain_for_duration : [valid_state < 0.5 && ...
      |  enable_gain]
  hold_gain_for_duration -> fade_gain : [hold_timer > hold_dur_msec]
  fade_gain -> (junction 25)
  data: enable_gain input; fading_gain input; hold_dur_msec input; valid_state input; gain output; hold_timer local; Ts parameter

== stateflow chart LSSFunctionLibrary/Delay_Reset/Sustain_wo_reset ==
  settings: description=_GWMH9P4.LKAFN.111_8_
  state Hold
    en:sustain_value = input;
    du:i=i+P_LCC_Ts;
    settings: description=_GWMH9P4.LKAFN.111_35_
  state Standby
    en:
    i=0;
    du:
    sustain_value = 0;
    settings: description=_GWMH9P4.LKAFN.111_36_
  (default) -> Standby
  Standby -> Hold : [input]
  Hold -> Hold [order 1] : [input]
      | {i=0;}
  Hold -> Standby [order 2] : [(i>= sustain_time) && (!input)]
  data: input input; sustain_time input; sustain_value output single; i local single; P_LCC_Ts parameter
  data input settings: description=_GWMH9P4.LKAFN.111_71_
  data sustain_time settings: description=_GWMH9P4.LKAFN.111_72_
  data sustain_value settings: description=_GWMAB30P4.LKAFN.111_83_
  data i settings: description=_GWMAB30P4.LKAFN.111_85_
